simulink model "LQR_FeedBackRegulation_EstimatedPlant"  (R2018a)
settings: Solver=VariableStepAuto  StartTime=0.0  StopTime=100  RelTol=1e-3
values from neighbouring files (symbols this model uses):
  A_Obs_est = A_est-L*C_est    [LQR_FeedBackRegulation.m]    (also in LQR_SetPoint_Regulation.m)
  B_Obs_est = [B_est-L*D_est L]    [LQR_FeedBackRegulation.m]    (also in LQR_SetPoint_Regulation.m)
  C_Obs_est = eye(4)    [LQR_FeedBackRegulation.m]    (also in LQR_SetPoint_Regulation.m)
  D_Obs_est = zeros(4,2)    [LQR_FeedBackRegulation.m]    (also in LQR_SetPoint_Regulation.m)
  k1 = (G_w0*W_np1^(2)*W_np2^(2))/(W_nz^(2))    [Esitmating_Plant_TF.m]    (also in LQR_FeedBackRegulation.m = K(1); LQR_SetPoint_Regulation.m = K(1); sineSweepOnVirtualPlant.m)
  k2 = K(2)    [LQR_FeedBackRegulation.m]    (also in LQR_SetPoint_Regulation.m)
  k3 = K(3)    [LQR_FeedBackRegulation.m]    (also in LQR_SetPoint_Regulation.m)
  k4 = K(4)    [LQR_FeedBackRegulation.m]    (also in LQR_SetPoint_Regulation.m)
  X0_est = randn(4,1)    [LQR_FeedBackRegulation.m]    (also in LQR_SetPoint_Regulation.m)
  X0_Obs = [0 0 0 0]'    [LQR_FeedBackRegulation.m]    (also in LQR_SetPoint_Regulation.m)
undefined symbols (not defined in the file or in its folder): A_est, B_est, C_est, D_est
settings Model: Creator=Dhruv  LastModifiedBy=ninadgaikwad
settings DataIOCC: SaveFinalState=on  SaveFormat=Structure  SaveState=on

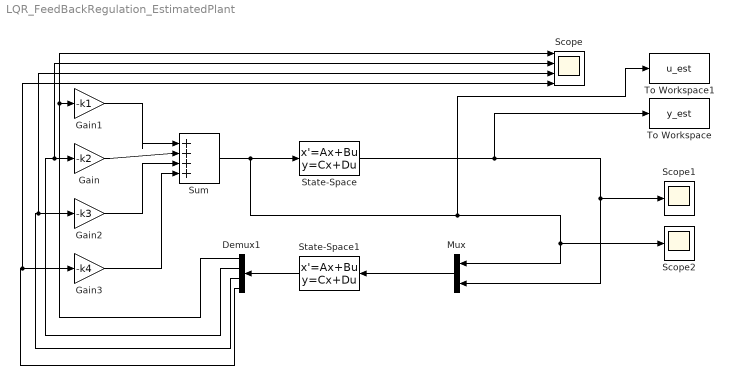
== system LQR_FeedBackRegulation_EstimatedPlant ==
  Demux1 : Demux
  Gain : Gain  Gain=-k2
  Gain1 : Gain  Gain=-k1
  Gain2 : Gain  Gain=-k3
  Gain3 : Gain  Gain=-k4
  Mux : Mux  Inputs=2
  Scope : Scope  NumInputPorts=4
  Scope1 : Scope
  Scope2 : Scope
  State-Space : StateSpace  A=A_est  B=B_est  C=C_est  D=D_est  InitialCondition=X0_est  ContinuousStateAttributes='Estimated_Plant'
  State-Space1 : StateSpace  A=A_Obs_est  B=B_Obs_est  C=C_Obs_est  D=D_Obs_est  InitialCondition=X0_Obs  ContinuousStateAttributes='Observer'
  Sum : Sum  Inputs=|++++
  To Workspace : ToWorkspace  VariableName=y_est  SampleTime=-1
  To Workspace1 : ToWorkspace  VariableName=u_est  SampleTime=-1
  wires:
  Mux/1 -> State-Space1/1
  State-Space/1 -> To Workspace/1, Scope1/1, Mux/2
  State-Space1/1 -> Demux1/1
  Sum/1 -> Scope2/1, Mux/1, To Workspace1/1, State-Space/1
  Gain1/1 -> Sum/1
  Gain/1 -> Sum/2
  Gain2/1 -> Sum/3
  Gain3/1 -> Sum/4
  Demux1/1 -> Scope/1, Gain1/1
  Demux1/2 -> Scope/2, Gain/1
  Demux1/4 -> Scope/4, Gain3/1
  Demux1/3 -> Scope/3, Gain2/1
